simulink model "SimuBFContinuDiscret_2020a"  (R2023b)
settings: Solver=VariableStepAuto  StartTime=0.0  StopTime=30  FixedStep=0.001  RelTol=1e-3
values from neighbouring files (symbols this model uses):
  A0 = 5.075    [script_param_s7.m]
  den = [1 0]    [script_param_s7.m]
  den_d = [1 -1]    [script_param_s7.m]
  den_sys = [2.328 1]    [script_param_s7.m]
  echelon = 1    [script_param_s7.m]
  fs = 100    [script_param_s7.m]
  num = [6.3 2.7027]    [script_param_s7.m]
  num_d = [6.314 -6.286]    [script_param_s7.m]
  u0 = 1    [script_param_s7.m]
  wn = 100    [script.m]    (also in script_param_s7.m = 40)
  y0 = 5.782    [script_param_s7.m]
  zeta = 0.7    [script.m]    (also in script_param_s7.m)
settings Model: Creator=Admin  LastModifiedBy=lucasp
settings SolverCC: AlgebraicLoopSolver=TrustRegion
settings DebuggingCC: UnconnectedInputMsg=warning  UnconnectedOutputMsg=warning  UnconnectedLineMsg=warning
settings ModelReferenceCC: EnableRefExpFcnMdlSchedulingChecks=on

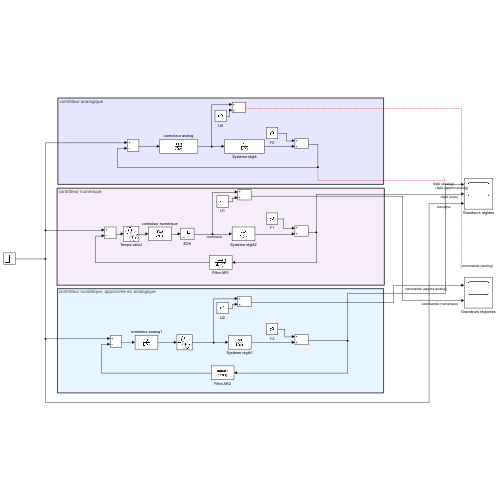
[thumbnail: Simulink's stored preview of the top-level diagram]
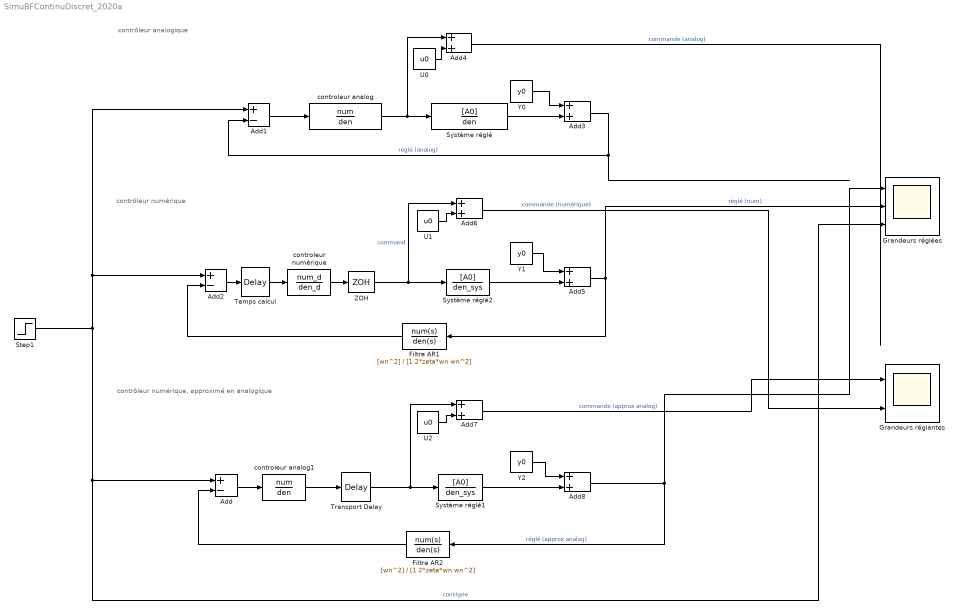
== system SimuBFContinuDiscret_2020a ==
  note: contrôleur numérique, approximé en analogique
  note: contrôleur numérique
  note: contrôleur analogique
  Add : Sum  Inputs=+-
  Add1 : Sum  Inputs=+-
  Add2 : Sum  Inputs=+-
  Add{3..8} (6 alike) : Sum
  Filtre AR1 : TransferFcn  Numerator=[wn^2]  Denominator=[1 2*zeta*wn wn^2]
  Filtre AR2 : TransferFcn  Numerator=[wn^2]  Denominator=[1 2*zeta*wn wn^2]
  Grandeurs réglantes : Scope  NumInputPorts=2
  Grandeurs réglées : Scope  NumInputPorts=3
  Step1 : Step  Time=10  Before=y0  After=y0+echelon  SampleTime=0
  Système réglé : TransferFcn  Numerator=[A0]  Denominator=den
  Système réglé1 : TransferFcn  Numerator=[A0]  Denominator=den_sys
  Système réglé2 : TransferFcn  Numerator=[A0]  Denominator=den_sys
  Temps calcul : TransportDelay  DelayTime=1/(2*fs)
  Transport Delay : TransportDelay  DelayTime=1/fs
  U0 : Constant  Value=u0
  U1 : Constant  Value=u0
  U2 : Constant  Value=u0
  Y0 : Constant  Value=y0
  Y1 : Constant  Value=y0
  Y2 : Constant  Value=y0
  ZOH : ZeroOrderHold  SampleTime=1/fs
  controleur analog : TransferFcn  Numerator=num  Denominator=den
  controleur analog1 : TransferFcn  Numerator=num  Denominator=den
  controleur numérique : DiscreteTransferFcn  Numerator=num_d  Denominator=den_d  SampleTime=1/fs
  wires:
  Add1/1 -> controleur analog/1
  controleur analog/1 -> Add4/1, Système réglé/1
  ZOH/1 -> Système réglé2/1, Add6/1  "command"
  controleur numérique/1 -> ZOH/1
  Add2/1 -> Temps calcul/1
  Système réglé/1 -> Add3/2
  Filtre AR1/1 -> Add2/2
  Temps calcul/1 -> controleur numérique/1
  controleur analog1/1 -> Transport Delay/1
  Transport Delay/1 -> Système réglé1/1, Add7/1
  Add/1 -> controleur analog1/1
  Filtre AR2/1 -> Add/2
  Step1/1 -> Grandeurs réglées/3, Add/1, Add1/1, Add2/1  "consigne"
  Système réglé1/1 -> Add8/2
  Système réglé2/1 -> Add5/2
  Add3/1 -> Add1/2  "réglé (analog)"
  Y0/1 -> Add3/1
  U0/1 -> Add4/2
  Add4/1 -> ?  "commande (analog)"
  Add5/1 -> Grandeurs réglées/2, Filtre AR1/1  "réglé (num)"
  Y1/1 -> Add5/1
  U1/1 -> Add6/2
  Add6/1 -> Grandeurs réglantes/2  "commande (numérique)"
  U2/1 -> Add7/2
  Add7/1 -> Grandeurs réglantes/1  "commande (approx analog)"
  Add8/1 -> Grandeurs réglées/1, Filtre AR2/1  "réglé (approx analog)"
  Y2/1 -> Add8/1
